simulink model "Example"  (R2019b)
settings: Solver=VariableStepAuto  StartTime=0.0  StopTime=100  RelTol=1e-3
libraries: ForceSeatDI_Simulink x2
settings Model: EnablePacing=on  Creator=usr  LastModifiedBy=usr

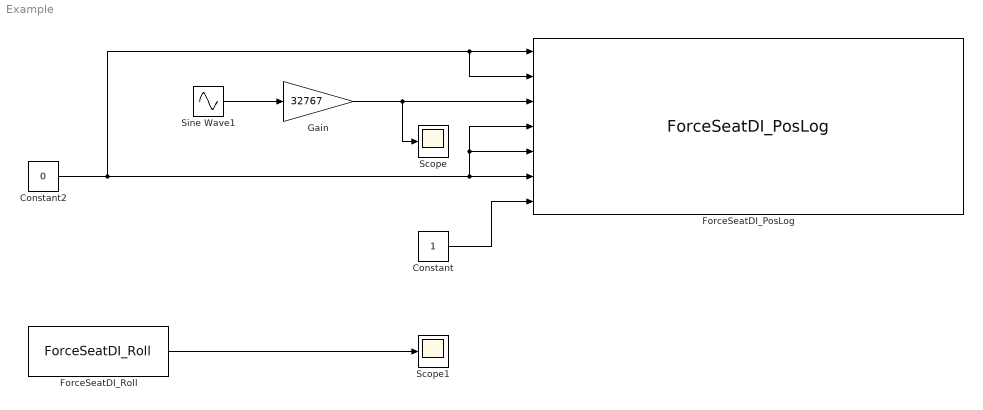
== system Example ==
  Constant : Constant  OutDataTypeStr=int32
  Constant2 : Constant  Value=0
  ForceSeatDI_PosLog : ForceSeatDI_Simulink/ForceSeatDI_PosLog
      settings: SourceProductName=MotionsSystems ForceSeatDI
  ForceSeatDI_Roll : ForceSeatDI_Simulink/ForceSeatDI_Roll
      settings: SourceProductName=MotionsSystems ForceSeatDI
  Gain : Gain  Gain=32767
  Scope : Scope
  Scope1 : Scope
  Sine Wave1 : Sin  SampleTime=0.01
  wires:
  Constant/1 -> ForceSeatDI_PosLog/7
  Constant2/1 -> ForceSeatDI_PosLog/6, ForceSeatDI_PosLog/4, ForceSeatDI_PosLog/5, ForceSeatDI_PosLog/1, ForceSeatDI_PosLog/2
  Gain/1 -> ForceSeatDI_PosLog/3, Scope/1
  Sine Wave1/1 -> Gain/1
  ForceSeatDI_Roll/1 -> Scope1/1
